simulink model "synthese_sim_retour_etat"  (R2018b)
settings: Solver=VariableStepAuto  StartTime=0.0  StopTime=50  RelTol=1e-3
values from neighbouring files (symbols this model uses):
  A = [0 0 1; 0 -alpha1 0; 0 sig1 -alpha2]    [synthese.m]
  alpha1 = 1    [synthese.m]
  alpha2 = 100    [synthese.m]
  B = [0; sig0; 0]    [synthese.m]
  C = [1 0 0]    [synthese.m]
  Fobs = Fe(1:3)    [synthese.m]
  Hobs = -Fe(4)    [synthese.m]
  L = acker(A', C',P)'    [synthese.m]
  sig0 = 1    [synthese.m]
  sig1 = 100    [synthese.m]
settings Model: Creator=poteaum  LastModifiedBy=poteaum

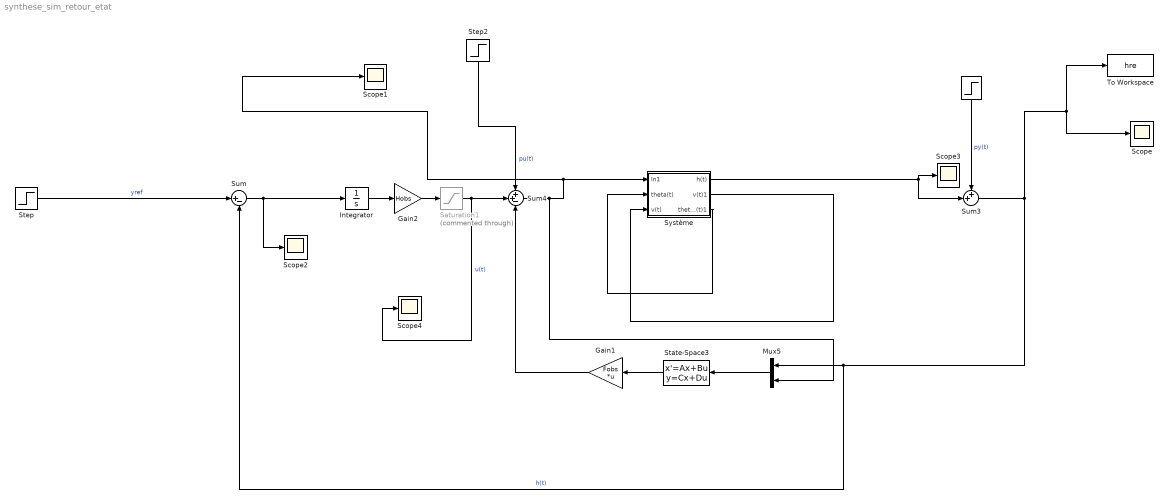
== system synthese_sim_retour_etat ==
  " " : Step  Time=10  After=0.1  SampleTime=0
  Gain1 : Gain  Gain=Fobs  Multiplication=Matrix(K*u)
  Gain2 : Gain  Gain=Hobs
  Integrator : Integrator
  Mux5 : Mux  Inputs=2
  Saturation1 : Saturate  Commented=through  UpperLimit=10  LowerLimit=-10
  Scope{,1..4} (5 alike) : Scope
  State-Space3 : StateSpace  A=A-L*C  B=[L B]  C=eye(3)  D=zeros(3,2)  InitialCondition=[0.1;0.1;0.1]
  Step : Step  Time=0  SampleTime=0
  Step2 : Step  Time=0  After=0.1  SampleTime=0
  Sum : Sum  Inputs=|+-
  Sum3 : Sum  Inputs=++|
  Sum4 : Sum  Inputs=++-
  Système : Subsystem
  To Workspace : ToWorkspace  VariableName=hre  SaveFormat=Structure With Time  SampleTime=-1
  wires:
  Sum/1 -> Scope2/1, Integrator/1
  Step/1 -> Sum/1  "yref"
  " "/1 -> Sum3/1  "py(t)"
  Sum3/1 -> Sum/2, Mux5/1, Scope/1, To Workspace/1  "h(t)"
  Step2/1 -> Sum4/1  "pu(t)"
  Système/2(v(t)1) -> Système/3(v(t))
  Système/1(h(t)) -> Sum3/2, Scope3/1
  Système/3(theta(t)1) -> Système/2(theta(t))
  Sum4/1 -> Mux5/2, Système/1(In1), Scope1/1
  State-Space3/1 -> Gain1/1
  Mux5/1 -> State-Space3/1
  Gain2/1 -> Saturation1/1
  Gain1/1 -> Sum4/3
  Integrator/1 -> Gain2/1
  Saturation1/1 -> Scope4/1, Sum4/2  "u(t)"

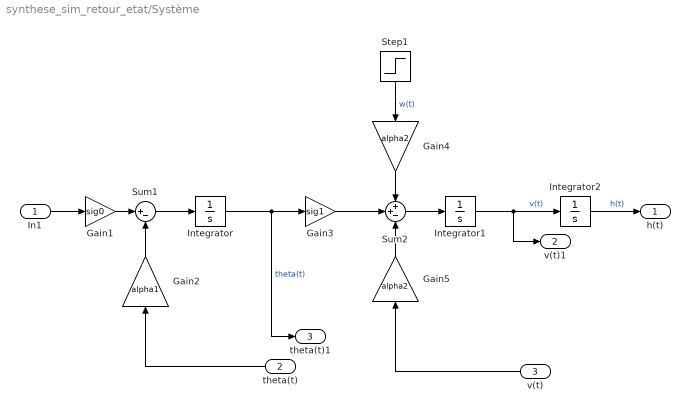
== system synthese_sim_retour_etat/Système ==
  In1 : Inport
  theta(t) : Inport  Port=2
  v(t) : Inport  Port=3
  Gain1 : Gain  Gain=sig0
  Gain2 : Gain  Gain=alpha1
  Gain3 : Gain  Gain=sig1
  Gain4 : Gain  Gain=alpha2
  Gain5 : Gain  Gain=alpha2
  Integrator : Integrator
  Integrator1 : Integrator
  Integrator2 : Integrator
  Step1 : Step  Time=0  After=0.01  SampleTime=0
  Sum1 : Sum  Inputs=|+-
  Sum2 : Sum  Inputs=++-
  h(t) : Outport
  v(t)1 : Outport  Port=2
  theta(t)1 : Outport  Port=3
  wires:
  Gain2/1 -> Sum1/2
  Gain4/1 -> Sum2/1
  In1/1 -> Gain1/1
  v(t)/1 -> Gain5/1
  Sum2/1 -> Integrator1/1
  Gain5/1 -> Sum2/3
  Integrator1/1 -> v(t)1/1, Integrator2/1  "v(t)"
  Gain1/1 -> Sum1/1
  Sum1/1 -> Integrator/1
  Step1/1 -> Gain4/1  "w(t)"
  Integrator/1 -> theta(t)1/1, Gain3/1  "theta(t)"
  theta(t)/1 -> Gain2/1
  Gain3/1 -> Sum2/2
  Integrator2/1 -> h(t)/1  "h(t)"
